simulink model "space_state"  (R2020b)
settings: Solver=VariableStepAuto  StartTime=0.0  StopTime=5  RelTol=1e-3
values from neighbouring files (symbols this model uses):
  A1 = [ ... (first row only)    [script_exp8.m]
  A2 = [ ... (first row only)    [script_exp8.m]
  B1 = [0 -m*g*d/L/(J/R^2+m)]'    [script_exp8.m]
  B2 = [0 0 0 1]'    [script_exp8.m]
  C1 = [1 0]    [script_exp8.m]
  C2 = [1 0 0 0]    [script_exp8.m]
  K1 = K1(1:2)    [script_exp8.m]
  K2 = K2(1:4)    [script_exp8.m]
  Ki1 = -K1(3)    [script_exp8.m]
  Ki2 = -K2(5)    [script_exp8.m]
  x10 = [0 0]'    [script_exp8.m]
  x20 = [0 0 0 0]'    [script_exp8.m]
  xi10 = 0    [script_exp8.m]
  xi20 = 0    [script_exp8.m]
settings Model: Creator=lucas  LastModifiedBy=lucas

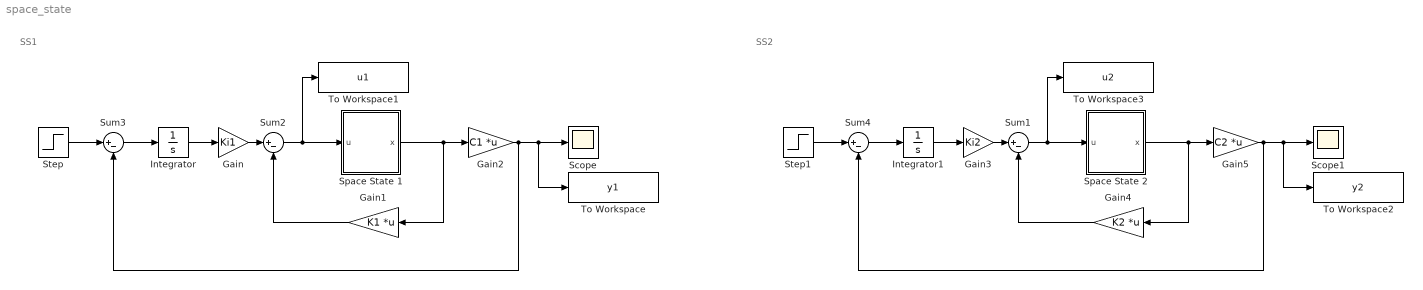
== system space_state ==
  note: SS1
  note: SS2
  Gain : Gain  Gain=Ki1
  Gain1 : Gain  Gain=K1  Multiplication=Matrix(K*u)
  Gain2 : Gain  Gain=C1  Multiplication=Matrix(K*u)
  Gain3 : Gain  Gain=Ki2
  Gain4 : Gain  Gain=K2  Multiplication=Matrix(K*u)
  Gain5 : Gain  Gain=C2  Multiplication=Matrix(K*u)
  Integrator : Integrator  InitialCondition=xi10
  Integrator1 : Integrator  InitialCondition=xi20
  Scope : Scope
  Scope1 : Scope
  Space State 1 : Subsystem
  Space State 2 : Subsystem
  Step : Step  Time=0  SampleTime=0
  Step1 : Step  Time=0  SampleTime=0
  Sum{1..4} (4 alike) : Sum  Inputs=|+-
  To Workspace : ToWorkspace  VariableName=y1  SaveFormat=Timeseries  SampleTime=-1
  To Workspace1 : ToWorkspace  VariableName=u1  SaveFormat=Timeseries  SampleTime=-1
  To Workspace2 : ToWorkspace  VariableName=y2  SaveFormat=Timeseries  SampleTime=-1
  To Workspace3 : ToWorkspace  VariableName=u2  SaveFormat=Timeseries  SampleTime=-1
  wires:
  Space State 1/1(x) -> Gain1/1, Gain2/1
  Sum2/1 -> To Workspace1/1, Space State 1/1(u)
  Gain2/1 -> Sum3/2, To Workspace/1, Scope/1
  Gain1/1 -> Sum2/2
  Sum3/1 -> Integrator/1
  Integrator/1 -> Gain/1
  Gain/1 -> Sum2/1
  Step/1 -> Sum3/1
  Gain4/1 -> Sum1/2
  Sum1/1 -> To Workspace3/1, Space State 2/1(u)
  Gain3/1 -> Sum1/1
  Gain5/1 -> Sum4/2, To Workspace2/1, Scope1/1
  Step1/1 -> Sum4/1
  Sum4/1 -> Integrator1/1
  Integrator1/1 -> Gain3/1
  Space State 2/1(x) -> Gain4/1, Gain5/1

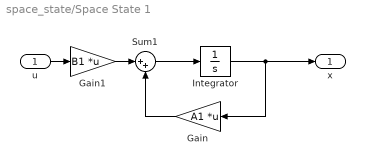
== system space_state/Space State 1 ==
  u : Inport
  Gain : Gain  Gain=A1  Multiplication=Matrix(K*u)
  Gain1 : Gain  Gain=B1  Multiplication=Matrix(K*u)
  Integrator : Integrator  InitialCondition=x10
  Sum1 : Sum  Inputs=|++
  x : Outport
  wires:
  Sum1/1 -> Integrator/1
  Gain1/1 -> Sum1/1
  Integrator/1 -> x/1, Gain/1
  u/1 -> Gain1/1
  Gain/1 -> Sum1/2

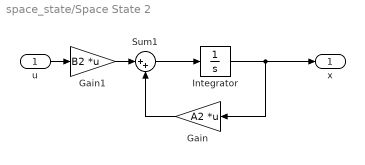
== system space_state/Space State 2 ==
  u : Inport
  Gain : Gain  Gain=A2  Multiplication=Matrix(K*u)
  Gain1 : Gain  Gain=B2  Multiplication=Matrix(K*u)
  Integrator : Integrator  InitialCondition=x20
  Sum1 : Sum  Inputs=|++
  x : Outport
  wires:
  Sum1/1 -> Integrator/1
  Gain1/1 -> Sum1/1
  Integrator/1 -> x/1, Gain/1
  u/1 -> Gain1/1
  Gain/1 -> Sum1/2
